simulink subsystem "GCS_in"  (R2024a)
settings: Solver=VariableStepAuto  StartTime=0.0  StopTime=10.0  RelTol=1e-3
libraries: dspnetwork x1
settings Model: Creator=gurt1  LastModifiedBy=gurt1

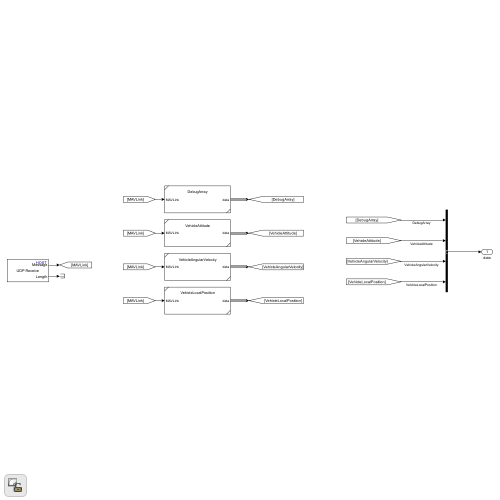
[thumbnail: Simulink's stored preview of the top-level diagram]
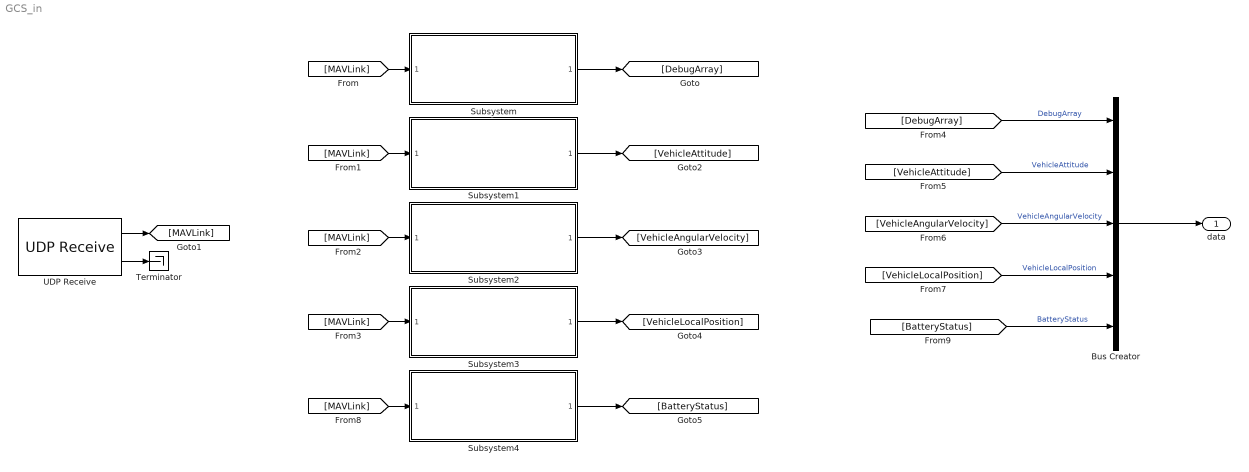
== system GCS_in ==
  Bus Creator : BusCreator  Inputs=5
  Subsystem : Subsystem  ReferencedSubsystem=DebugArray
  Subsystem1 : Subsystem  ReferencedSubsystem=VehicleAttitude
  Subsystem2 : Subsystem  ReferencedSubsystem=VehicleAngularVelocity
  Subsystem3 : Subsystem  ReferencedSubsystem=VehicleLocalPosition
  Subsystem4 : Subsystem  ReferencedSubsystem=BatteryStatus
  Terminator : Terminator
  UDP Receive : dspnetwork/UDP Receive  localURL='0.0.0.0'  localPort=14445  remoteURL='0.0.0.0'  remotePort=-1  recvBufferSize=8192  dims=512  signalDatatype=uint8  isComplex=off  isVarSize=off  showBlockingTime=on  blockingTime=0  sampletime=1/200  blockPlatform=HOST
      settings: LibrarySourceBlock=embeddedtargetslib/Host Communication/UDP Receive
  data : Outport
  wires:
  UDP Receive/1 -> [MAVLink]
  UDP Receive/2 -> Terminator/1
  [MAVLink] -> Subsystem/1
  Subsystem/1 -> [DebugArray]
  [MAVLink] -> Subsystem1/1
  Subsystem1/1 -> [VehicleAttitude]
  Subsystem2/1 -> [VehicleAngularVelocity]
  [MAVLink] -> Subsystem2/1
  [MAVLink] -> Subsystem3/1
  Subsystem3/1 -> [VehicleLocalPosition]
  [DebugArray] -> Bus Creator/1  "DebugArray"
  [VehicleAttitude] -> Bus Creator/2  "VehicleAttitude"
  [VehicleAngularVelocity] -> Bus Creator/3  "VehicleAngularVelocity"
  [VehicleLocalPosition] -> Bus Creator/4  "VehicleLocalPosition"
  Bus Creator/1 -> data/1
  Subsystem4/1 -> [BatteryStatus]
  [MAVLink] -> Subsystem4/1
  [BatteryStatus] -> Bus Creator/5  "BatteryStatus"
